simulink model "ver_2015b"  (R2015b)
settings: Solver=ode45  SolverMode=SingleTasking  StartTime=0.0  StopTime=1000  FixedStep=0.01  MaxStep=1  RelTol=1e-3
values from neighbouring files (symbols this model uses):
  A = [-0.026014706155  0  0; 0.032019398003  -0.0381052395202  0; 0  0.0262404235325  -0.0208551931358]    [matrix_A.mat]
  B = [4.13177021749 0 0]    [matrix_B.mat]
  C = eye(3)    [wywolanie_new.m]
  K = lqr(A, B, Q, R)    [wywolanie_new.m]
  L = lqe(A,G,C,Q,R)    [wywolanie_new.m]
undefined symbols (not defined in the file or in its folder): sol1, sol2, sol3, ur, x1r, x2r, x3r
settings Model: Creator=Student  LastModifiedBy=szczy
settings DataIOCC: SaveFormat=Array
settings DebuggingCC: AllowSymbolicDim=on
settings HardwareCC: ProdBitPerPointer=32  ProdLargestAtomicFloat=None  ProdIntDivRoundTo=Undefined  ProdEndianess=Unspecified  ProdWordSize=32  ProdHWDeviceType=32-bit Generic
settings ModelReferenceCC: EnableRefExpFcnMdlSchedulingChecks=off
settings ConfigComp: CovModelRefEnable=Off

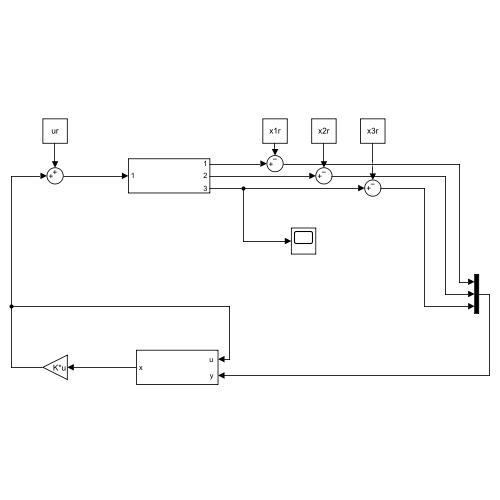
[thumbnail: Simulink's stored preview of the top-level diagram]
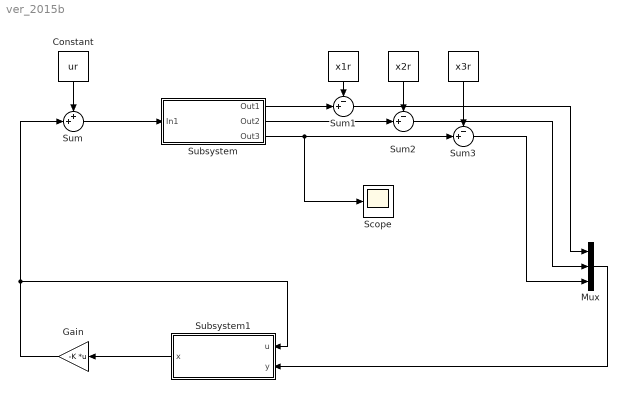
== system ver_2015b ==
  " " : Constant  Value=x2r
  " " : Constant  Value=x1r
  " " : Constant  Value=x3r
  Constant : Constant  Value=ur
  Gain : Gain  Gain=-K  Multiplication=Matrix(K*u)
  Mux : Mux  Inputs=3
  Scope : Scope
  Subsystem : Subsystem
  Subsystem1 : Subsystem
  Sum : Sum  Inputs=++|
  Sum1 : Sum  Inputs=-+|
  Sum2 : Sum  Inputs=-+|
  Sum3 : Sum  Inputs=-+|
  wires:
  Subsystem/1(Out1) -> Sum1/2
  Subsystem1/1(x) -> Gain/1
  Gain/1 -> Subsystem1/1("u "), Sum/2
  " "/1 -> Sum1/1
  Constant/1 -> Sum/1
  Subsystem/2(Out2) -> Sum2/2
  Subsystem/3(Out3) -> Scope/1, Sum3/2
  " "/1 -> Sum2/1
  " "/1 -> Sum3/1
  Sum2/1 -> Mux/2
  Sum3/1 -> Mux/3
  Sum1/1 -> Mux/1
  Mux/1 -> Subsystem1/2("y ")
  Sum/1 -> Subsystem/1(In1)

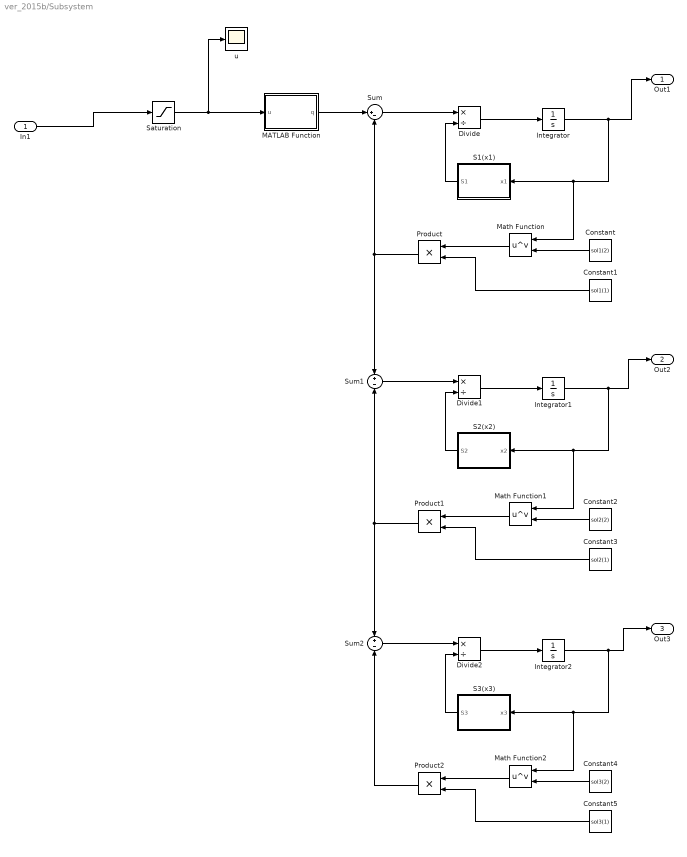
== system ver_2015b/Subsystem ==
  In1 : Inport
  Constant : Constant  Value=sol1(2)
  Constant1 : Constant  Value=sol1(1)
  Constant2 : Constant  Value=sol2(2)
  Constant3 : Constant  Value=sol2(1)
  Constant4 : Constant  Value=sol3(2)
  Constant5 : Constant  Value=sol3(1)
  Divide : Product  Inputs=*/
  Divide1 : Product  Inputs=*/
  Divide2 : Product  Inputs=*/
  Integrator : Integrator  InitialCondition=x1r  LimitOutput=on  LowerSaturationLimit=0.1
  Integrator1 : Integrator  InitialCondition=x2r  LimitOutput=on  LowerSaturationLimit=0.1
  Integrator2 : Integrator  InitialCondition=x3r-4  LimitOutput=on  LowerSaturationLimit=0.1
  MATLAB Function : MATLAB Function  TreatAsAtomicUnit=on
  Math Function : Math  Operator=pow  SaturateOnIntegerOverflow=on
  Math Function1 : Math  Operator=pow  SaturateOnIntegerOverflow=on
  Math Function2 : Math  Operator=pow  SaturateOnIntegerOverflow=on
  Product : Product
  Product1 : Product
  Product2 : Product
  S1(x1) : MATLAB Function  TreatAsAtomicUnit=on
  S2(x2) : MATLAB Function  TreatAsAtomicUnit=on
  S3(x3) : MATLAB Function  TreatAsAtomicUnit=on
  Saturation : Saturate  UpperLimit=1  LowerLimit=0.5
  Sum : Sum  Inputs=|+-
  Sum1 : Sum  Inputs=+-
  Sum2 : Sum  Inputs=+-
  u : Scope
  Out1 : Outport
  Out2 : Outport  Port=2
  Out3 : Outport  Port=3
  wires:
  Saturation/1 -> MATLAB Function/1(u), u/1
  MATLAB Function/1(q) -> Sum/1
  Sum/1 -> Divide/1
  S1(x1)/1(S1) -> Divide/2
  Divide/1 -> Integrator/1
  Integrator/1 -> Math Function/1, S1(x1)/1(x1), Out1/1
  Constant/1 -> Math Function/2
  Math Function/1 -> Product/1
  Constant1/1 -> Product/2
  Product/1 -> Sum/2, Sum1/1
  Sum1/1 -> Divide1/1
  S2(x2)/1(S2) -> Divide1/2
  Divide1/1 -> Integrator1/1
  Integrator1/1 -> Math Function1/1, S2(x2)/1(x2), Out2/1
  Constant2/1 -> Math Function1/2
  Math Function1/1 -> Product1/1
  Constant3/1 -> Product1/2
  Product1/1 -> Sum2/1, Sum1/2
  Sum2/1 -> Divide2/1
  S3(x3)/1(S3) -> Divide2/2
  Divide2/1 -> Integrator2/1
  Integrator2/1 -> Math Function2/1, S3(x3)/1(x3), Out3/1
  Constant4/1 -> Math Function2/2
  Math Function2/1 -> Product2/1
  Constant5/1 -> Product2/2
  Product2/1 -> Sum2/2
  In1/1 -> Saturation/1

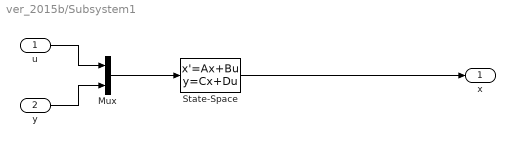
== system ver_2015b/Subsystem1 ==
  "u " : Inport
  "y " : Inport  Port=2
  Mux : Mux  Inputs=2
  State-Space : StateSpace  A=A-L*C  B=[B L]  C=eye(3)  D=zeros(3,4)  X0=zeros(3,1)
  x : Outport
  wires:
  "u "/1 -> Mux/1
  "y "/1 -> Mux/2
  Mux/1 -> State-Space/1
  State-Space/1 -> x/1

== matlab function ver_2015b/Subsystem/S1(x1) ==
  data: x1 input; S1 output
function S1 = fcn(x1)
a = 10.5;
b = 35.8;
c = 25;
w = 3.4;
H = 25;
R = 36.5;
S1 = c*w;

== matlab function ver_2015b/Subsystem/MATLAB Function ==
  data: u input; q output
function q = fcn(u)
a = -231.6274;
b = 625.0864;
c = -254.4828;
q = a*(u^2) + b*u + c;

== matlab function ver_2015b/Subsystem/S2(x2) ==
  data: x2 input; S2 output
function S2 = fcn(x2)
a = 10.5;
b = 35.8;
w = 3.4;
H = 25;
S2 = w*(((b-a)/H)*x2 + a);

== matlab function ver_2015b/Subsystem/S3(x3) ==
  data: x3 input; S3 output
function S3 = fcn(x3)
a = 10.5;
b = 35.8;
c = 25;
w = 3.4;
H = 25;
R = 36.5;
S3 = w*sqrt(2*R*x3 - x3^2);
